simulink model "project8allprts"  (R2017a)
settings: Solver=ode4  StartTime=0  StopTime=60  FixedStep=0.01  RelTol=1e-3  EnableMultiTasking=on
undefined symbols (not defined in the file or in its folder): mc
settings Model: Creator=Jinesh  LastModifiedBy=Jinesh

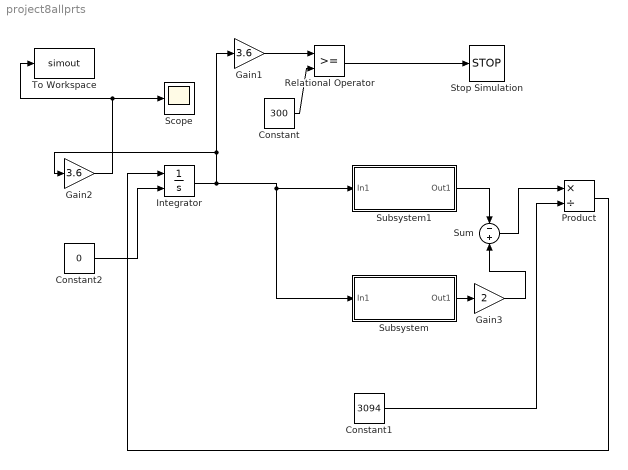
== system project8allprts ==
  Constant : Constant  Value=300
  Constant1 : Constant  Value=3094
  Constant2 : Constant  Value=0
  Gain1 : Gain  Gain=3.6
  Gain2 : Gain  Gain=3.6
  Gain3 : Gain  Gain=2
  Integrator : Integrator  InitialConditionSource=external
  Product : Product  Inputs=*/
  Relational Operator : RelationalOperator  OutDataTypeStr=boolean  RndMeth=Simplest
  Scope : Scope
  Stop Simulation : Stop
  Subsystem : Subsystem
  Subsystem1 : Subsystem
  Sum : Sum  Inputs=-+
  To Workspace : ToWorkspace  VariableName=simout  SaveFormat=Timeseries  SampleTime=-1
  wires:
  Subsystem1/1(Out1) -> Sum/1
  Subsystem/1(Out1) -> Gain3/1
  Gain3/1 -> Sum/2
  Sum/1 -> Product/1
  Constant1/1 -> Product/2
  Constant2/1 -> Integrator/2
  Product/1 -> Integrator/1
  Integrator/1 -> Gain1/1, Gain2/1, Subsystem/1(In1), Subsystem1/1(In1)
  Constant/1 -> Relational Operator/2
  Relational Operator/1 -> Stop Simulation/1
  Gain1/1 -> Relational Operator/1
  Gain2/1 -> Scope/1, To Workspace/1

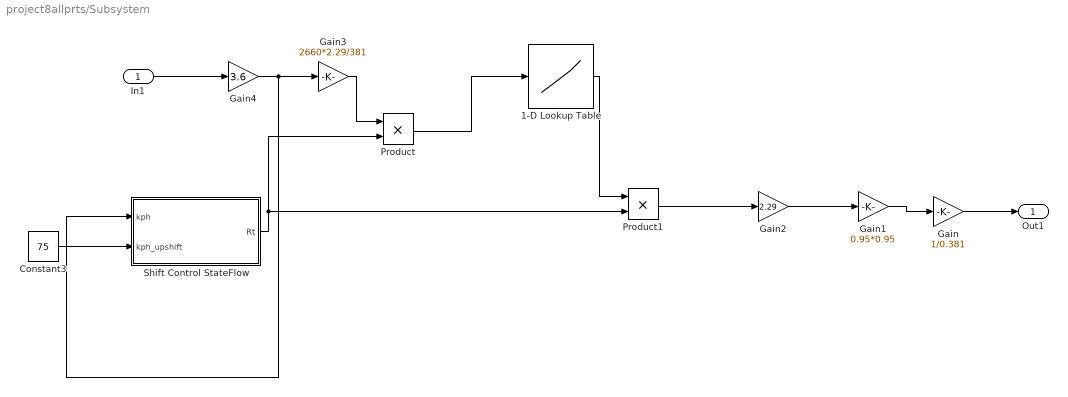
== system project8allprts/Subsystem ==
  In1 : Inport
  1-D Lookup Table : Lookup_n-D  NumberOfTableDimensions=1  BreakpointsForDimension1=mc.rpm_max_index  Table=mc.trq_max_map  InternalRulePriority=Speed  RndMeth=Simplest  InputSameDT=on
  Constant3 : Constant  Value=75
  Gain : Gain  Gain=1/0.381
  Gain1 : Gain  Gain=0.95*0.95
  Gain2 : Gain  Gain=2.29
  Gain3 : Gain  Gain=2660*2.29/381
  Gain4 : Gain  Gain=3.6
  Product : Product
  Product1 : Product
  Shift Control StateFlow : Stateflow chart  TreatAsAtomicUnit=on
  Out1 : Outport
  wires:
  Gain3/1 -> Product/1
  1-D Lookup Table/1 -> Product1/1
  Gain2/1 -> Gain1/1
  Gain1/1 -> Gain/1
  Gain/1 -> Out1/1
  Gain4/1 -> Gain3/1, Shift Control StateFlow/1(kph)
  In1/1 -> Gain4/1
  Constant3/1 -> Shift Control StateFlow/2(kph_upshift)
  Shift Control StateFlow/1(Rt) -> Product/2, Product1/2
  Product/1 -> 1-D Lookup Table/1
  Product1/1 -> Gain2/1

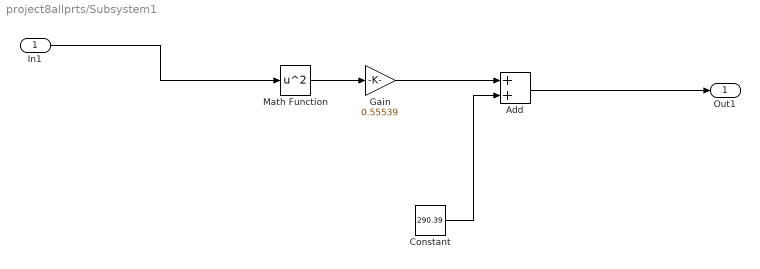
== system project8allprts/Subsystem1 ==
  In1 : Inport
  Add : Sum
  Constant : Constant  Value=290.39
  Gain : Gain  Gain=0.55539
  Math Function : Math  Operator=square  SaturateOnIntegerOverflow=on
  Out1 : Outport
  wires:
  In1/1 -> Math Function/1
  Math Function/1 -> Gain/1
  Gain/1 -> Add/1
  Constant/1 -> Add/2
  Add/1 -> Out1/1

== stateflow chart project8allprts/Subsystem/Shift Control StateFlow ==
  state first_gear
    entry: Rt = 5;
  state second_gear
    entry: Rt = 2.5
  (default) -> first_gear
  first_gear -> second_gear : [kph>kph_upshift]
  second_gear -> first_gear : [kph<kph_upshift-5]
  data: kph input; Rt output double; kph_upshift input
